simulink model "model_5LinkWalk_NODS_soft_ground"  (R2022b)
settings: Solver=VariableStepAuto  StartTime=0.0  StopTime=Tf  FixedStep=1e-5  MaxStep=1e-3  RelTol=1e-12  AbsTol=1e-8
values from neighbouring files (symbols this model uses):
  gains = [K_p,K_d,K_p,K_d,K_p,K_d,K_p,K_d,K_p,K_d]    [main_soft_ground.m]
  init_flag = [-1; 0; ocl_traj.x_sw(1); init_t_mode_change; alpha_ref(1); 0; y_g_curr]    [main_soft_ground.m]
  Initial_state = [q0;dq0]    [main_soft_ground.m]
  joint_angles_ref = [ocl_traj.time, ocl_traj.simout, alpha_ref]    [main_soft_ground.m]
  landing_ref = [landing_traj.time, landing_traj.simout, alpha_ref_landing]    [main_soft_ground.m]
  param = [ ... (first row only)    [main_soft_ground.m]
  sample_time = time(2) - time(1)    [animation_floating.m]    (also in main_soft_ground.m = 0.001)
undefined symbols (not defined in the file or in its folder): uneven_terrain
libraries: simulink x2
(part 2 of 2)

== matlab function model_5LinkWalk_NODS_soft_ground/Model dynamics/Mode Changer/Mode Changer 5Link ==
  data: X_minus input; flag output; flag_minus input; param input; uneven_terrain input; joint_angles_ref input; X_reset output; time input
function [flag, X_reset]  = fcn(X_minus, flag_minus, param, uneven_terrain, joint_angles_ref, time)

%% variables

x_st = X_minus(1);
y_st = X_minus(2);
th1 = X_minus(3);
th2 = X_minus(4);
th3 = X_minus(5);
th4 = X_minus(6);
th5 = X_minus(7);

dx_st = X_minus(8);
dy_st = X_minus(9);
dth1 = X_minus(10);
dth2 = X_minus(11);
dth3 = X_minus(12);
dth4 = X_minus(13);
dth5 = X_minus(14);

q = [x_st;y_st;th1;th2;th3;th4;th5];
dq = [dx_st;dy_st;dth1;dth2;dth3;dth4;dth5];

%% parameters

m1 = param(1);
m2 = param(2);
m3 = m2;
m4 = m1;
m5 = param(3);

l1 = param(4);
l2 = param(5);
l5 = param(6);
l3 = l2;
l4 = l1;

gravi = param(7);
I1 = param(8);
I2 = param(9);
I5 = param(10);
I3 = I1;
I4 = I2;

q_minus = q;
dq_minus = dq;

%% flags
f_impact = flag_minus(1); % indicates which stance phase it is
foot_x = flag_minus(2); % location of the stance foot
foot_x_prev = flag_minus(3); % previous location of the stance foot
t_LO = flag_minus(4); % previous location of the stance foot
alpha_TD = flag_minus(5); % x_CoM location when liftOff happens
f_alpha_ob = flag_minus(6); % alpha is out of bounds flag
foot_y = flag_minus(7); 

%% reference 
alpha_ref = joint_angles_ref(:,12);

%%
X_reset = [q_minus; dq_minus]; % dummy X_reset so that simulink doesn't give error

%% calculating the Swing foot position and velocity
Psw_tip_minus = [x_st + l1*cos(th1) + l2*cos(th1 + th2) + l3*cos(th1 + th2 + th3) + l4*cos(th1 + th2 + th3 + th4);
                 y_st + l1*sin(th1) + l2*sin(th1 + th2) + l3*sin(th1 + th2 + th3) + l4*sin(th1 + th2 + th3 + th4)];

J_Psw_tip_minus = [1, 0, - l4*sin(th1 + th2 + th3 + th4) - l2*sin(th1 + th2) - l1*sin(th1) - l3*sin(th1 + th2 + th3), - l4*sin(th1 + th2 + th3 + th4) - l2*sin(th1 + th2) - l3*sin(th1 + th2 + th3), - l4*sin(th1 + th2 + th3 + th4) - l3*sin(th1 + th2 + th3), -l4*sin(th1 + th2 + th3 + th4), 0;
                   0, 1, l4*cos(th1 + th2 + th3 + th4) + l2*cos(th1 + th2) + l1*cos(th1) + l3*cos(th1 + th2 + th3),   l4*cos(th1 + th2 + th3 + th4) + l2*cos(th1 + th2) + l3*cos(th1 + th2 + th3),   l4*cos(th1 + th2 + th3 + th4) + l3*cos(th1 + th2 + th3),  l4*cos(th1 + th2 + th3 + th4), 0];

dPsw_tip_minus = J_Psw_tip_minus*dq_minus;

%% DS constraint equations
% obtained from derive_EoM_relative_floating.m

J_c_impact = [
    1, 0, - l4*sin(th1 + th2 + th3 + th4) - l2*sin(th1 + th2) - l1*sin(th1) - l3*sin(th1 + th2 + th3), - l4*sin(th1 + th2 + th3 + th4) - l2*sin(th1 + th2) - l3*sin(th1 + th2 + th3), - l4*sin(th1 + th2 + th3 + th4) - l3*sin(th1 + th2 + th3), -l4*sin(th1 + th2 + th3 + th4), 0];


%% calculating the current height of the ground (uneven ground)
x_sw = Psw_tip_minus(1,1);
x_ground = uneven_terrain.track_start:uneven_terrain.dist_step_size:uneven_terrain.track_end;
y_ground = uneven_terrain.y_g_curr;
y_ground_curr = interp1(x_ground, y_ground, foot_x + x_sw);


%%

% if f_SS == 1 && Psw_tip_minus(2,1) <= 0.005 && dPsw_tip_minus(2,1) < -0.5
if Psw_tip_minus(2,1) <= y_ground_curr && dPsw_tip_minus(2,1) < -0.005 && f_impact ~= 1
    % touchdown (impact)
    f_impact = 1;
    foot_x_prev = foot_x; % saving the old foot location
    foot_x = Psw_tip_minus(1,1); % calculating the new foots location
    foot_y = y_ground_curr; % new stance foot height
           
    % Impact mapによる衝突後の状態の計算
    MM_minus = [m1 + m2 + m3 + m4 + m5, 0, - (m3*(2*l2*sin(th1 + th2) + 2*l1*sin(th1) + l3*sin(th1 + th2 + th3)))/2 - (m5*(2*l2*sin(th1 + th2) + 2*l1*sin(th1) + l5*sin(th1 + th2 + th5)))/2 - (m2*(l2*sin(th1 + th2) + 2*l1*sin(th1)))/2 - (m4*(l4*sin(th1 + th2 + th3 + th4) + 2*l2*sin(th1 + th2) + 2*l1*sin(th1) + 2*l3*sin(th1 + th2 + th3)))/2 - (l1*m1*sin(th1))/2, - (m4*(l4*sin(th1 + th2 + th3 + th4) + 2*l2*sin(th1 + th2) + 2*l3*sin(th1 + th2 + th3)))/2 - (m3*(2*l2*sin(th1 + th2) + l3*sin(th1 + th2 + th3)))/2 - (m5*(2*l2*sin(th1 + th2) + l5*sin(th1 + th2 + th5)))/2 - (l2*m2*sin(th1 + th2))/2, - (m4*(l4*sin(th1 + th2 + th3 + th4) + 2*l3*sin(th1 + th2 + th3)))/2 - (l3*m3*sin(th1 + th2 + th3))/2, -(l4*m4*sin(th1 + th2 + th3 + th4))/2, -(l5*m5*sin(th1 + th2 + th5))/2; 0, m1 + m2 + m3 + m4 + m5, (m3*(2*l2*cos(th1 + th2) + 2*l1*cos(th1) + l3*cos(th1 + th2 + th3)))/2 + (m5*(2*l2*cos(th1 + th2) + 2*l1*cos(th1) + l5*cos(th1 + th2 + th5)))/2 + (m2*(l2*cos(th1 + th2) + 2*l1*cos(th1)))/2 + (m4*(l4*cos(th1 + th2 + th3 + th4) + 2*l2*cos(th1 + th2) + 2*l1*cos(th1) + 2*l3*cos(th1 + th2 + th3)))/2 + (l1*m1*cos(th1))/2, (m3*(2*l2*cos(th1 + th2) + l3*cos(th1 + th2 + th3)))/2 + (m5*(2*l2*cos(th1 + th2) + l5*cos(th1 + th2 + th5)))/2 + (m4*(l4*cos(th1 + th2 + th3 + th4) + 2*l2*cos(th1 + th2) + 2*l3*cos(th1 + th2 + th3)))/2 + (l2*m2*cos(th1 + th2))/2, (m4*(l4*cos(th1 + th2 + th3 + th4) + 2*l3*cos(th1 + th2 + th3)))/2 + (l3*m3*cos(th1 + th2 + th3))/2, (l4*m4*cos(th1 + th2 + th3 + th4))/2, (l5*m5*cos(th1 + th2 + th5))/2; - (m3*(2*l2*sin(th1 + th2) + 2*l1*sin(th1) + l3*sin(th1 + th2 + th3)))/2 - (m5*(2*l2*sin(th1 + th2) + 2*l1*sin(th1) + l5*sin(th1 + th2 + th5)))/2 - (m2*(l2*sin(th1 + th2) + 2*l1*sin(th1)))/2 - (m4*(l4*sin(th1 + th2 + th3 + th4) + 2*l2*sin(th1 + th2) + 2*l1*sin(th1) + 2*l3*sin(th1 + th2 + th3)))/2 - (l1*m1*sin(th1))/2, (m3*(2*l2*cos(th1 + th2) + 2*l1*cos(th1) + l3*cos(th1 + th2 + th3)))/2 + (m5*(2*l2*cos(th1 + th2) + 2*l1*cos(th1) + l5*cos(th1 + th2 + th5)))/2 + (m2*(l2*cos(th1 + th2) + 2*l1*cos(th1)))/2 + (m4*(l4*cos(th1 + th2 + th3 + th4) + 2*l2*cos(th1 + th2) + 2*l1*cos(th1) + 2*l3*cos(th1 + th2 + th3)))/2 + (l1*m1*cos(th1))/2, I1 + I2 + I3 + I4 + I5 + (l1^2*m1)/4 + l1^2*m2 + l1^2*m3 + (l2^2*m2)/4 + l1^2*m4 + l2^2*m3 + l1^2*m5 + l2^2*m4 + (l3^2*m3)/4 + l2^2*m5 + l3^2*m4 + (l4^2*m4)/4 + (l5^2*m5)/4 + l1*l3*m3*cos(th2 + th3) + 2*l1*l3*m4*cos(th2 + th3) + l2*l4*m4*cos(th3 + th4) + l1*l5*m5*cos(th2 + th5) + l1*l2*m2*cos(th2) + 2*l1*l2*m3*cos(th2) + 2*l1*l2*m4*cos(th2) + 2*l1*l2*m5*cos(th2) + l2*l3*m3*cos(th3) + 2*l2*l3*m4*cos(th3) + l3*l4*m4*cos(th4) + l2*l5*m5*cos(th5) + l1*l4*m4*cos(th2 + th3 + th4), I2 + I3 + I4 + I5 + (l2^2*m2)/4 + l2^2*m3 + l2^2*m4 + (l3^2*m3)/4 + l2^2*m5 + l3^2*m4 + (l4^2*m4)/4 + (l5^2*m5)/4 + (l1*l3*m3*cos(th2 + th3))/2 + l1*l3*m4*cos(th2 + th3) + l2*l4*m4*cos(th3 + th4) + (l1*l5*m5*cos(th2 + th5))/2 + (l1*l2*m2*cos(th2))/2 + l1*l2*m3*cos(th2) + l1*l2*m4*cos(th2) + l1*l2*m5*cos(th2) + l2*l3*m3*cos(th3) + 2*l2*l3*m4*cos(th3) + l3*l4*m4*cos(th4) + l2*l5*m5*cos(th5) + (l1*l4*m4*cos(th2 + th3 + th4))/2, I3 + I4 + (l3^2*m3)/4 + l3^2*m4 + (l4^2*m4)/4 + (l1*l3*m3*cos(th2 + th3))/2 + l1*l3*m4*cos(th2 + th3) + (l2*l4*m4*cos(th3 + th4))/2 + (l2*l3*m3*cos(th3))/2 + l2*l3*m4*cos(th3) + l3*l4*m4*cos(th4) + (l1*l4*m4*cos(th2 + th3 + th4))/2, I4 + (l4^2*m4)/4 + (l2*l4*m4*cos(th3 + th4))/2 + (l3*l4*m4*cos(th4))/2 + (l1*l4*m4*cos(th2 + th3 + th4))/2, I5 + (l5^2*m5)/4 + (l1*l5*m5*cos(th2 + th5))/2 + (l2*l5*m5*cos(th5))/2; - (m4*(l4*sin(th1 + th2 + th3 + th4) + 2*l2*sin(th1 + th2) + 2*l3*sin(th1 + th2 + th3)))/2 - (m3*(2*l2*sin(th1 + th2) + l3*sin(th1 + th2 + th3)))/2 - (m5*(2*l2*sin(th1 + th2) + l5*sin(th1 + th2 + th5)))/2 - (l2*m2*sin(th1 + th2))/2, (m3*(2*l2*cos(th1 + th2) + l3*cos(th1 + th2 + th3)))/2 + (m5*(2*l2*cos(th1 + th2) + l5*cos(th1 + th2 + th5)))/2 + (m4*(l4*cos(th1 + th2 + th3 + th4) + 2*l2*cos(th1 + th2) + 2*l3*cos(th1 + th2 + th3)))/2 + (l2*m2*cos(th1 + th2))/2, I2 + I3 + I4 + I5 + (l2^2*m2)/4 + l2^2*m3 + l2^2*m4 + (l3^2*m3)/4 + l2^2*m5 + l3^2*m4 + (l4^2*m4)/4 + (l5^2*m5)/4 + (l1*l3*m3*cos(th2 + th3))/2 + l1*l3*m4*cos(th2 + th3) + l2*l4*m4*cos(th3 + th4) + (l1*l5*m5*cos(th2 + th5))/2 + (l1*l2*m2*cos(th2))/2 + l1*l2*m3*cos(th2) + l1*l2*m4*cos(th2) + l1*l2*m5*cos(th2) + l2*l3*m3*cos(th3) + 2*l2*l3*m4*cos(th3) + l3*l4*m4*cos(th4) + l2*l5*m5*cos(th5) + (l1*l4*m4*cos(th2 + th3 + th4))/2, I2 + I3 + I4 + I5 + (l2^2*m2)/4 + l2^2*m3 + l2^2*m4 + (l3^2*m3)/4 + l2^2*m5 + l3^2*m4 + (l4^2*m4)/4 + (l5^2*m5)/4 + l2*l4*m4*cos(th3 + th4) + l2*l3*m3*cos(th3) + 2*l2*l3*m4*cos(th3) + l3*l4*m4*cos(th4) + l2*l5*m5*cos(th5), I3 + I4 + (l3^2*m3)/4 + l3^2*m4 + (l4^2*m4)/4 + (l2*l4*m4*cos(th3 + th4))/2 + (l2*l3*m3*cos(th3))/2 + l2*l3*m4*cos(th3) + l3*l4*m4*cos(th4), I4 + (l4^2*m4)/4 + (l2*l4*m4*cos(th3 + th4))/2 + (l3*l4*m4*cos(th4))/2, I5 + (l5^2*m5)/4 + (l2*l5*m5*cos(th5))/2; - (m4*(l4*sin(th1 + th2 + th3 + th4) + 2*l3*sin(th1 + th2 + th3)))/2 - (l3*m3*sin(th1 + th2 + th3))/2, (m4*(l4*cos(th1 + th2 + th3 + th4) + 2*l3*cos(th1 + th2 + th3)))/2 + (l3*m3*cos(th1 + th2 + th3))/2, I3 + I4 + (l3^2*m3)/4 + l3^2*m4 + (l4^2*m4)/4 + (l1*l3*m3*cos(th2 + th3))/2 + l1*l3*m4*cos(th2 + th3) + (l2*l4*m4*cos(th3 + th4))/2 + (l2*l3*m3*cos(th3))/2 + l2*l3*m4*cos(th3) + l3*l4*m4*cos(th4) + (l1*l4*m4*cos(th2 + th3 + th4))/2, I3 + I4 + (l3^2*m3)/4 + l3^2*m4 + (l4^2*m4)/4 + (l2*l4*m4*cos(th3 + th4))/2 + (l2*l3*m3*cos(th3))/2 + l2*l3*m4*cos(th3) + l3*l4*m4*cos(th4), I3 + I4 + (l3^2*m3)/4 + l3^2*m4 + (l4^2*m4)/4 + l3*l4*m4*cos(th4), I4 + (l4^2*m4)/4 + (l3*l4*m4*cos(th4))/2, 0; -(l4*m4*sin(th1 + th2 + th3 + th4))/2, (l4*m4*cos(th1 + th2 + th3 + th4))/2, I4 + (l4^2*m4)/4 + (l2*l4*m4*cos(th3 + th4))/2 + (l3*l4*m4*cos(th4))/2 + (l1*l4*m4*cos(th2 + th3 + th4))/2, I4 + (l4^2*m4)/4 + (l2*l4*m4*cos(th3 + th4))/2 + (l3*l4*m4*cos(th4))/2, I4 + (l4^2*m4)/4 + (l3*l4*m4*cos(th4))/2, I4 + (l4^2*m4)/4, 0; -(l5*m5*sin(th1 + th2 + th5))/2, (l5*m5*cos(th1 + th2 + th5))/2, I5 + (l5^2*m5)/4 + (l1*l5*m5*cos(th2 + th5))/2 + (l2*l5*m5*cos(th5))/2, I5 + (l5^2*m5)/4 + (l2*l5*m5*cos(th5))/2, 0, 0, I5 + (l5^2*m5)/4];
    dq_after = (eye(7)-inv(MM_minus)*J_c_impact'*inv(J_c_impact*inv(MM_minus)*J_c_impact')*J_c_impact)*dq_minus;
    
    %
    x_st_after = Psw_tip_minus(1,1);
    y_st_after = Psw_tip_minus(2,1);
    th1_after = q_minus(6,1) + q_minus(5,1) + q_minus(4,1) + q_minus(3,1) - pi; % th1 becomes th4
    th2_after = - q_minus(6,1); % th2 becomes th3
    th3_after = - q_minus(5,1); % th3 becomes th2
    th4_after = - q_minus(4,1); % th4 becomes th1
    %th5_after = q_minus(5,1) - q_minus(3,1) + pi;
    th5_after = q_minus(3,1) + q_minus(4,1) + q_minus(7,1) - (th1_after + th2_after);
    
    % constraining angles to pi 2pi
    th1_after = mod(th1_after, 2*pi);
    th2_after = mod(th2_after, 2*pi);
    th3_after = mod(th3_after, 2*pi) - 2*pi;
    th4_after = mod(th4_after, 2*pi);
    th5_after = th5_after - 2*pi;
    
    q_after = [x_st_after; y_st_after; th1_after; th2_after; th3_after; th4_after; th5_after]; % this is where the switching happens
    
    dx_st_after = dq_after(1,1);
    dy_st_after = dq_after(2,1);
    dth1_after = dq_after(6,1) + dq_after(5,1) + dq_after(4,1) + dq_after(3,1); % th1 becomes th4
    dth2_after = - dq_after(6,1); % th2 becomes th3
    dth3_after = - dq_after(5,1); % th3 becomes th2
    dth4_after = - dq_after(4,1); % th4 becomes th1
    dth5_after = dq_after(7,1) - dq_after(5,1);
    
    dq_after = [dx_st_after; dy_st_after; dth1_after; dth2_after; dth3_after; dth4_after; dth5_after];

    % Reset state if the f_ss change from 1 to 0 (from single stance to
    % double stance)
    X_reset = [q_after; dq_after];
    
    alpha_TD = pi - (2*th1_after + th2_after)/2;
    t_LO = time;
    
    % check is alpha is out of bounds and raise the flag is so
    if alpha_TD < alpha_ref(1)
        f_alpha_ob = 1;
    else
        f_alpha_ob = 0;
    end
        
elseif f_impact == 1 && Psw_tip_minus(2,1) > y_ground_curr + 0.01
    f_impact = -1;

end

flag = [f_impact; foot_x; foot_x_prev; t_LO; alpha_TD; f_alpha_ob; foot_y];

== matlab function model_5LinkWalk_NODS_soft_ground/Model dynamics/STOP system when dx_CoM<=0/MATLAB Function2 ==
  data: X input; param input; flag input; flag_zCoM_pos output; flag_xCoM_vel output; flag_th2 output; flag_th4 output; flag_5 output
function [flag_zCoM_pos, flag_xCoM_vel, flag_th2, flag_th4, flag_5] = fcn(X,param, flag)

%% variables
x_st = X(1);
y_st = X(2);
th1 = X(3);
th2 = X(4);
th3 = X(5);
th4 = X(6);
th5 = X(7);

dx_st = X(8);
dy_st = X(9);
dth1 = X(10);
dth2 = X(11);
dth3 = X(12);
dth4 = X(13);
dth5 = X(14);

%% parameters

m1 = param(1);
m2 = param(2);
m3 = m2;
m4 = m1;
m5 = param(3);

l1 = param(4);
l2 = param(5);
l5 = param(6);
l3 = l2;
l4 = l1;

gravi = param(7);
I1 = param(8);
I2 = param(9);
I5 = param(10);
I3 = I1;
I4 = I2;

k_s = param(11);
r_k = param(12);
r_b = param(13);

%% flags
f_SS = flag(1); % indicates which stance phase it is
foot = flag(2); % location of the stance foot
foot_prev = flag(3); % previous location of the stance foot

%% CoM calculation
% CoM = [xG, zG, dxG, dzG, ddxG, ddzG];
X_non_floating = [th1;th2;th3;th4;th5;dth1;dth2;dth3;dth4;dth5];
CoM = calculate_com(X_non_floating, param, flag, [0;0;0;0;0]); % calculation the CoM location

xG = CoM(1);
zG = CoM(2);
dxG = CoM(3);
dzG = CoM(4);

%%

% flag_zCoM_pos: if z_CoM drops or rises above certain value
flag_zCoM_pos = 0;
if zG >= 1.5
    flag_zCoM_pos = 1;
elseif zG <= 0.7
    flag_zCoM_pos = 1;
end

% flag_xCoM_vel
flag_xCoM_vel = 0;
if dxG <= 0
    flag_xCoM_vel = 1;
end

% flag_th2
flag_th2 = 0;
if mod(th2,2*pi) <= 0
    flag_th2 = 1;
end

% flag_th4
flag_th4 = 0;
if mod(th4,2*pi) >= 0
%     flag_th4 = 1;
end

% flag_th5
flag_5 = 0;
if foot > 0
    flag_5 = 0;
end
